simulink model "sim_projet"  (R2022a)
settings: Solver=VariableStepAuto  StartTime=0.0  StopTime=20  RelTol=1e-3
settings Model: Creator=kckel  LastModifiedBy=kckel

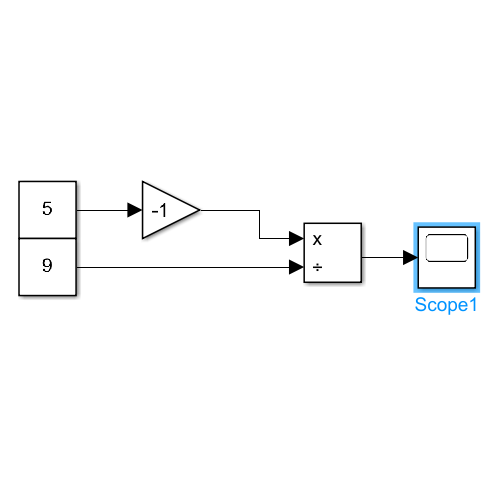
[thumbnail: Simulink's stored preview of the top-level diagram]
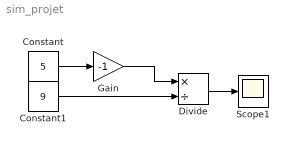
== system sim_projet ==
  Constant : Constant  Value=5
  Constant1 : Constant  Value=9
  Divide : Product  Inputs=*/
  Gain : Gain  Gain=-1
  Scope1 : Scope
  wires:
  Gain/1 -> Divide/1
  Constant/1 -> Gain/1
  Constant1/1 -> Divide/2
  Divide/1 -> Scope1/1
